simulink model "ex00_model"  (R2023a)
settings: Solver=FixedStepDiscrete  StartTime=0.0  StopTime=1  RelTol=1e-3
values from neighbouring files (symbols this model uses):
  Fc = 125e3    (= 125000)    [ex00.m]    (also in ex00_config.m; ex01.m = 62500; ex01_config.m = 62500; ex02.m)
  fir_num = fir1(fir_ord, Wn, hann(fir_ord+1))    [ex00.m]    (also in ex00_config.m; ex01.m; ex01_config.m; ex02.m)
  L = 4    [ex00.m]    (also in ex00_config.m; ex02.m = 5; ex02_config.m = 5)
  Ts = 1/Fs    (= 1e-06)    [ex00.m]    (also in ex00_config.m; ex01.m; ex01_config.m; ex02.m)
libraries: dspsrcs4 x2, dspsigops x1
settings Model: Creator=daniele  LastModifiedBy=daniele

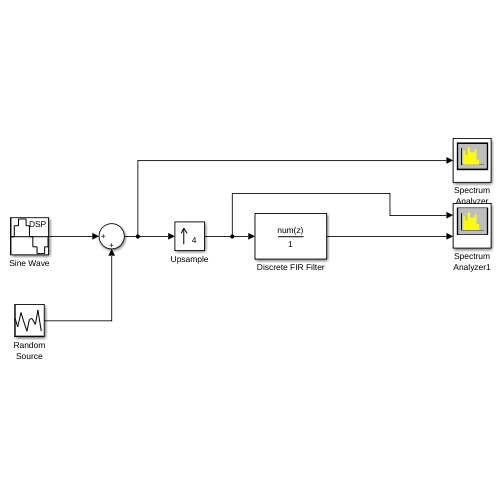
[thumbnail: Simulink's stored preview of the top-level diagram]
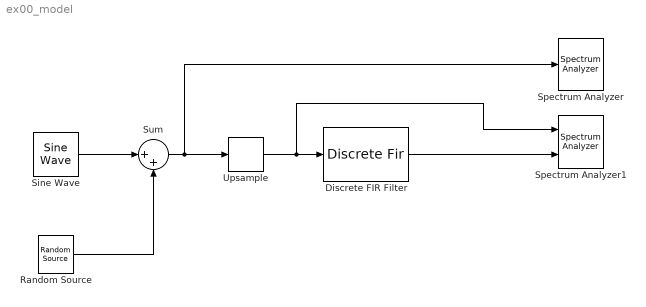
== system ex00_model ==
  Discrete FIR Filter : DiscreteFir  Coefficients=fir_num
  Random Source : dspsrcs4/Random Source  SrcType=Gaussian  NormMethod=Ziggurat  CltLength=12  MinVal=0  MaxVal=1  MeanVal=0  VarVal=0.1  RepMode=Not repeatable  rawSeed=1  IsInherit=off  SampMode=Discrete  SampTime=Ts  SampFrame=1  DataType=Double  OutComplex=Real  OutputFrames=off
  Sine Wave : dspsrcs4/Sine Wave  Amplitude=1  Frequency=Fc  Phase=pi/2  SampleMode=Discrete  OutComplex=Real  CompMethod=Trigonometric fcn  TableSize=Speed  SampleTime=Ts  SamplesPerFrame=1  ResetState=Restart at time zero  OutputFrames=off  dataType=double  wordLen=16  udDataType=sfix(16)  fracBitsMode=Best precision  numFracBits=15  OutDataTypeStr=double  LastOutDataTypeStr=double
  Spectrum Analyzer : SpectrumAnalyzer  WindowPosition=[186.000000,290.000000,800.000000,500.000000,]  ScopeFrameLocation=window  YLimits=[-18.33064242,28.65923266]  ColorLimits=[-20 80]  DefaultConfigurationName=spbscopes.SpectrumAnalyzerBlockCfg  IsFrequencyInputMode=0  FrequencyVectorPort=0  FrequencyVectorFromPort=0  FrequencyInputRBWPort=0  FrequencyInputRBWFromPort=0
  Spectrum Analyzer1 : SpectrumAnalyzer  NumInputPorts=2  WindowPosition=[956.000000,290.000000,800.000000,500.000000,]  ScopeFrameLocation=window  YLimits=[-167.4486866,31.87045355]  ColorLimits=[-20 80]  ShowLegend=on  DefaultConfigurationName=spbscopes.SpectrumAnalyzerBlockCfg  IsFrequencyInputMode=0  FrequencyVectorPort=0  FrequencyVectorFromPort=0  FrequencyInputRBWPort=0  FrequencyInputRBWFromPort=0
  Sum : Sum  Inputs=|++
  Upsample : dspsigops/Upsample  FactorSource=Dialog parameter  N=L  Nmax=16  phase=0  RateOptions=Allow multirate processing  ic=0  mode=Unused parameter value
      settings: LibrarySourceBlock=dsphdlsupportsigops/Upsample
  wires:
  Sine Wave/1 -> Sum/1
  Random Source/1 -> Sum/2
  Sum/1 -> Spectrum Analyzer/1, Upsample/1
  Upsample/1 -> Spectrum Analyzer1/1, Discrete FIR Filter/1
  Discrete FIR Filter/1 -> Spectrum Analyzer1/2
